simulink model "gm_uz_JL_invModel_PT1"  (R2025a)
settings: Solver=FixedStepDiscrete  StartTime=0.0  StopTime=10.0  RelTol=1e-3
settings Model: Creator=jonat  LastModifiedBy=jonat
settings SolverCC: AlgebraicLoopSolver=TrustRegion
settings DataIOCC: LimitDataPoints=on  SaveOutput=off  SaveTime=off
settings OptimizationCC: BlockReduction=off  ConditionallyExecuteInputs=off  DefaultParameterBehavior=Inlined  InheritOutputTypeSmallerThanSingle=on  LifeSpan=inf
settings DebuggingCC: AlgebraicLoopMsg=error  InheritedTsInSrcMsg=none  SingleTaskRateTransMsg=error  UnconnectedInputMsg=warning  UnconnectedOutputMsg=warning  UnconnectedLineMsg=warning  AllowSymbolicDim=off  StrictBusMsg=ErrorOnBusTreatedAsVector  SFUnexpectedBacktrackingDiag=warning  SFNoUnconditionalDefaultTransitionDiag=warning  SFExecutionAtInitializationDiag=none  ArithmeticOperatorsInVariantConditions=warning
settings HardwareCC: ProdBitPerPointer=32.0  ProdBitPerSizeT=32.0  ProdBitPerPtrDiffT=32.0  ProdLargestAtomicFloat=None  ProdIntDivRoundTo=Undefined  ProdEndianess=Unspecified  ProdWordSize=32.0  ProdHWDeviceType=ASIC/FPGA->ASIC/FPGA  ProdEqTarget=off
settings ModelReferenceCC: EnableRefExpFcnMdlSchedulingChecks=on
settings SFSimCC: SimUseLocalCustomCode=off  CustomCodeUndefinedFunction=UseInterfaceOnly
settings RTWCC: RTWUseLocalCustomCode=off  GPUComputeCapability=3.5
settings CodeAppCC: StateflowObjectComments=on
settings GRTTargetCC: TargetLangStandard=C89/C90 (ANSI)
settings ConfigComp: CovScope=ReferencedModels  CovMetricSettings=dw  CovSaveCumulativeToWorkspaceVar=on  CovSaveSingleToWorkspaceVar=on  CovExternalEMLEnable=off  CovSFcnEnable=off

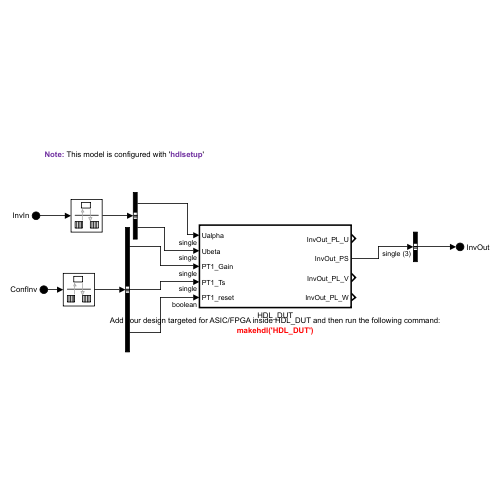
[thumbnail: Simulink's stored preview of the top-level diagram]
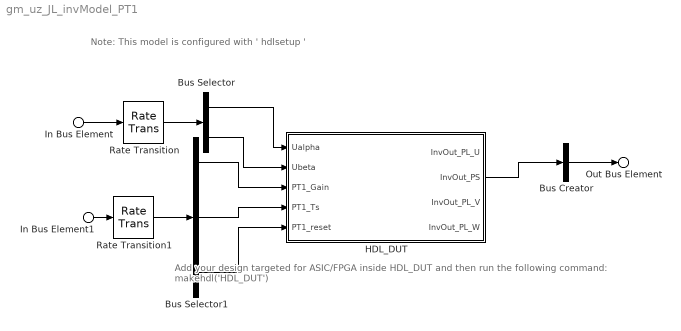
== system gm_uz_JL_invModel_PT1 ==
  note: Add your design targeted for ASIC/FPGA inside HDL_DUT and then run the following command:
      | makehdl('HDL_DUT')
  note: Note: This model is configured with ' hdlsetup '
  In Bus Element : Inport  PortName=InvIn
  In Bus Element1 : Inport  Port=2  PortName=ConfInv
  Bus Creator : BusCreator  Inputs=1  OutDataTypeStr=Bus: Bus_Inv_Out
      settings: InheritFromInputs=off
  Bus Selector : BusSelector  OutputSignals=Ualpha,Ubeta
  Bus Selector1 : BusSelector  OutputSignals=PT1_Gain,PT1_Ts,PT1_reset
  HDL_DUT : Subsystem  TreatAsAtomicUnit=on
  Rate Transition : RateTransition  OutPortSampleTime=1/1e6
  Rate Transition1 : RateTransition  OutPortSampleTime=1/1e6
  Out Bus Element : Outport  PortName=InvOut
  wires:
  Bus Selector1/3 -> HDL_DUT/5(PT1_reset)
  Bus Selector1/2 -> HDL_DUT/4(PT1_Ts)
  Bus Selector1/1 -> HDL_DUT/3(PT1_Gain)
  Bus Selector/2 -> HDL_DUT/2(Ubeta)
  Bus Selector/1 -> HDL_DUT/1(Ualpha)
  Bus Creator/1 -> Out Bus Element/1
  HDL_DUT/2(InvOut_PS) -> Bus Creator/1
  Rate Transition1/1 -> Bus Selector1/1
  Rate Transition/1 -> Bus Selector/1
  In Bus Element1/1 -> Rate Transition1/1
  In Bus Element/1 -> Rate Transition/1

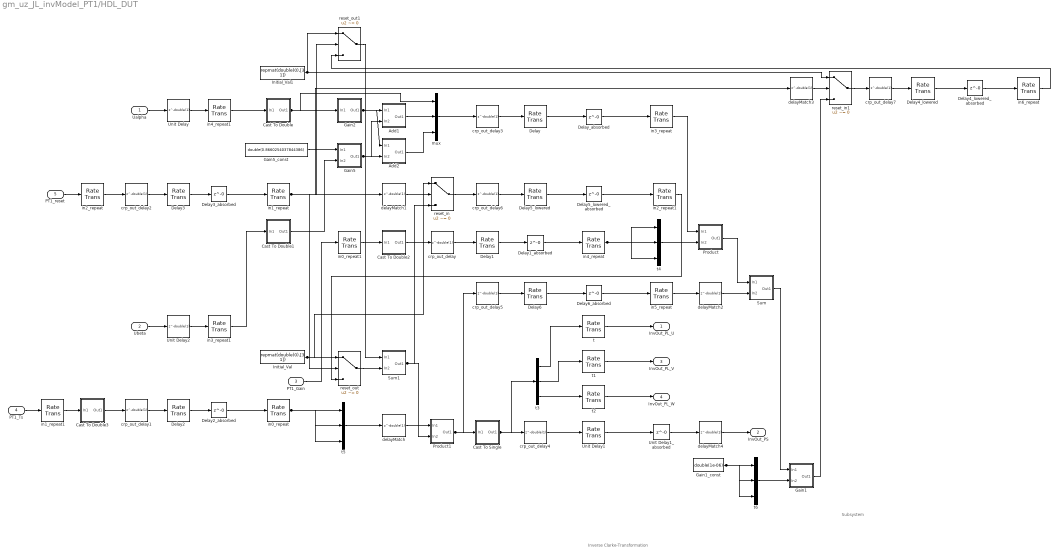
== system gm_uz_JL_invModel_PT1/HDL_DUT ==
  note: Subsystem
  note: Inverse Clarke-Transformation
  Ualpha : Inport  OutDataTypeStr=single  PortDimensions=1  SampleTime=1e-06
  Ubeta : Inport  Port=2  OutDataTypeStr=single  PortDimensions=1  SampleTime=1e-06
  PT1_Gain : Inport  Port=3  OutDataTypeStr=single  PortDimensions=1  SampleTime=1e-06
  PT1_Ts : Inport  Port=4  OutDataTypeStr=single  PortDimensions=1  SampleTime=1e-06
  PT1_reset : Inport  Port=5  OutDataTypeStr=boolean  PortDimensions=1  SampleTime=1e-06
  Add1 : Subsystem
      mask Display: disp('NFP\nadd');
  Add2 : Subsystem
      mask Display: disp('NFP\nadd');
  Cast To Double : Subsystem
      mask Display: disp('NFP\nconv');
  Cast To Double1 : Subsystem
      mask Display: disp('NFP\nconv');
  Cast To Double2 : Subsystem
      mask Display: disp('NFP\nconv');
  Cast To Double3 : Subsystem
      mask Display: disp('NFP\nconv');
  Cast To Single : Subsystem
      mask Display: disp('NFP\nconv');
  Delay{,1..3,6} (5 alike) : RateTransition  InitialCondition=double(0)  OutPortSampleTimeOpt=Multiple of input port sample time  OutPortSampleTimeMultiple=30
  Delay1_absorbed : Delay  DelayLength=0
  Delay2_absorbed : Delay  DelayLength=0
  Delay3_absorbed : Delay  DelayLength=0
  Delay4_lowered : RateTransition  InitialCondition=double(0)  OutPortSampleTimeOpt=Multiple of input port sample time  OutPortSampleTimeMultiple=30
  Delay4_lowered_absorbed : Delay  DelayLength=0
  Delay5_lowered : RateTransition  InitialCondition=double(0)  OutPortSampleTimeOpt=Multiple of input port sample time  OutPortSampleTimeMultiple=30
  Delay5_lowered_absorbed : Delay  DelayLength=0
  Delay6_absorbed : Delay  DelayLength=0
  Delay_absorbed : Delay  DelayLength=0
  Gain1 : Subsystem
      mask Display: disp('NFP\nmul');
  Gain1_const : Constant  Value=double(1e-06)  OutDataTypeStr=double  SampleTime=3.33333333333333e-08
  Gain2 : Subsystem
      mask Display: disp('NFP\ngain_pow2');
  Gain5 : Subsystem
      mask Display: disp('NFP\nmul');
  Gain5_const : Constant  Value=double(0.8660254037844386)  OutDataTypeStr=double  SampleTime=3.33333333333333e-08
  Initial_Val : Constant  Value="repmat(double(0),[3  1])"  OutDataTypeStr=double  SampleTime=3.33333333333333e-08
  Initial_Val1 : Constant  Value="repmat(double(0),[3  1])"  OutDataTypeStr=double  SampleTime=3.33333333333333e-08
  Product : Subsystem
      mask Display: disp('NFP\nmul');
  Product1 : Subsystem
      mask Display: disp('NFP\nmul');
  Sum : Subsystem
      mask Display: disp('NFP\nadd');
  Sum1 : Subsystem
      mask Display: disp('NFP\nadd');
  Unit Delay : Delay  DelayLength=double(1)  InitialCondition=0  SampleTime=1e-06
  Unit Delay1 : RateTransition  InitialCondition=double(0)  OutPortSampleTimeOpt=Multiple of input port sample time  OutPortSampleTimeMultiple=30
  Unit Delay1_absorbed : Delay  DelayLength=0
  Unit Delay2 : Delay  DelayLength=double(1)  InitialCondition=0  SampleTime=1e-06
  crp_out_delay{,1..7} (8 alike) : Delay  DelayLength=double(1)  InitialCondition=0  SampleTime=3.33333333333333e-08
  delayMatch{,1..3} (4 alike) : Delay  DelayLength=double(1)  InitialCondition=0  SampleTime=3.33333333333333e-08
  delayMatch4 : Delay  DelayLength=double(1)  InitialCondition=0  SampleTime=1e-06
  in0_repeat : RateTransition  Integrity=off  Deterministic=off  OutPortSampleTimeOpt=Multiple of input port sample time  OutPortSampleTimeMultiple=1/30
  in0_repeat1 : RateTransition  Integrity=off  Deterministic=off  OutPortSampleTimeOpt=Multiple of input port sample time  OutPortSampleTimeMultiple=1/30
  in1_repeat : RateTransition  Integrity=off  Deterministic=off  OutPortSampleTimeOpt=Multiple of input port sample time  OutPortSampleTimeMultiple=1/30
  in1_repeat1 : RateTransition  Integrity=off  Deterministic=off  OutPortSampleTimeOpt=Multiple of input port sample time  OutPortSampleTimeMultiple=1/30
  in2_repeat : RateTransition  Integrity=off  Deterministic=off  OutPortSampleTimeOpt=Multiple of input port sample time  OutPortSampleTimeMultiple=1/30
  in2_repeat1 : RateTransition  Integrity=off  Deterministic=off  OutPortSampleTimeOpt=Multiple of input port sample time  OutPortSampleTimeMultiple=1/30
  in3_repeat : RateTransition  Integrity=off  Deterministic=off  OutPortSampleTimeOpt=Multiple of input port sample time  OutPortSampleTimeMultiple=1/30
  in3_repeat1 : RateTransition  Integrity=off  Deterministic=off  OutPortSampleTimeOpt=Multiple of input port sample time  OutPortSampleTimeMultiple=1/30
  in4_repeat : RateTransition  Integrity=off  Deterministic=off  OutPortSampleTimeOpt=Multiple of input port sample time  OutPortSampleTimeMultiple=1/30
  in4_repeat1 : RateTransition  Integrity=off  Deterministic=off  OutPortSampleTimeOpt=Multiple of input port sample time  OutPortSampleTimeMultiple=1/30
  in5_repeat : RateTransition  Integrity=off  Deterministic=off  OutPortSampleTimeOpt=Multiple of input port sample time  OutPortSampleTimeMultiple=1/30
  in6_repeat : RateTransition  Integrity=off  Deterministic=off  OutPortSampleTimeOpt=Multiple of input port sample time  OutPortSampleTimeMultiple=1/30
  mux : Mux  Inputs=3
  reset_in : Switch  Criteria=u2 ~= 0  Threshold=double(0)  OutDataTypeStr=double  SampleTime=3.33333333333333e-08  SaturateOnIntegerOverflow=off  InputSameDT=off
  reset_in1 : Switch  Criteria=u2 ~= 0  Threshold=double(0)  OutDataTypeStr=double  SampleTime=3.33333333333333e-08  SaturateOnIntegerOverflow=off  InputSameDT=off
  reset_out : Switch  Criteria=u2 ~= 0  Threshold=double(0)  OutDataTypeStr=double  SampleTime=3.33333333333333e-08  SaturateOnIntegerOverflow=off  InputSameDT=off
  reset_out1 : Switch  Criteria=u2 ~= 0  Threshold=double(0)  OutDataTypeStr=double  SampleTime=3.33333333333333e-08  SaturateOnIntegerOverflow=off  InputSameDT=off
  t : RateTransition  InitialCondition=double(0)  OutPortSampleTimeOpt=Multiple of input port sample time  OutPortSampleTimeMultiple=30
  t1 : RateTransition  InitialCondition=double(0)  OutPortSampleTimeOpt=Multiple of input port sample time  OutPortSampleTimeMultiple=30
  t2 : RateTransition  InitialCondition=double(0)  OutPortSampleTimeOpt=Multiple of input port sample time  OutPortSampleTimeMultiple=30
  t3 : Demux  Outputs=3
  t4 : Mux  Inputs=3
  t5 : Mux  Inputs=3
  t6 : Mux  Inputs=3
  InvOut_PL_U : Outport  SampleTime=1e-06
  InvOut_PS : Outport  Port=2  SampleTime=1e-06
  InvOut_PL_V : Outport  Port=3  SampleTime=1e-06
  InvOut_PL_W : Outport  Port=4  SampleTime=1e-06
  wires:
  Delay/1 -> Delay_absorbed/1
  delayMatch/1 -> Product1/1(In1)
  reset_out/1 -> Sum1/2(In2)
  in1_repeat/1 -> delayMatch3/1, delayMatch1/1, reset_out1/2, reset_out/2
  PT1_Ts/1 -> in1_repeat1/1
  PT1_reset/1 -> in2_repeat/1
  crp_out_delay5/1 -> Delay6/1
  Delay5_lowered_absorbed/1 -> in2_repeat1/1
  in1_repeat1/1 -> Cast To Double3/1(In1)
  crp_out_delay6/1 -> Delay5_lowered/1
  crp_out_delay2/1 -> Delay3/1
  Delay6_absorbed/1 -> in5_repeat/1
  Gain5/1(Out1) -> Add1/2(In2), Add2/2(In2)
  Initial_Val1/1 -> reset_in1/1, reset_out1/1
  in2_repeat/1 -> crp_out_delay2/1
  Cast To Double3/1(Out1) -> crp_out_delay1/1
  Gain5_const/1 -> Gain5/1(In1)
  Ubeta/1 -> Unit Delay2/1
  reset_out1/1 -> Sum1/1(In1)
  Ualpha/1 -> Unit Delay/1
  crp_out_delay1/1 -> Delay2/1
  Delay2/1 -> Delay2_absorbed/1
  Unit Delay/1 -> in4_repeat1/1
  crp_out_delay3/1 -> Delay/1
  delayMatch1/1 -> reset_in/2
  Delay3/1 -> Delay3_absorbed/1
  crp_out_delay7/1 -> Delay4_lowered/1
  in0_repeat/1 -> t5/3, t5/2, t5/1
  Unit Delay2/1 -> in3_repeat1/1
  Delay_absorbed/1 -> in3_repeat/1
  in4_repeat1/1 -> Cast To Double/1(In1)
  Delay3_absorbed/1 -> in1_repeat/1
  in3_repeat1/1 -> Cast To Double1/1(In1)
  Delay2_absorbed/1 -> in0_repeat/1
  Cast To Double/1(Out1) -> Gain2/1(In1), mux/1
  mux/1 -> crp_out_delay3/1
  Cast To Double1/1(Out1) -> Gain5/2(In2)
  Cast To Double2/1(Out1) -> crp_out_delay/1
  t5/1 -> delayMatch/1
  Initial_Val/1 -> reset_in/1, reset_out/1
  Delay1/1 -> Delay1_absorbed/1
  reset_in/1 -> crp_out_delay6/1
  PT1_Gain/1 -> in0_repeat1/1
  Gain2/1(Out1) -> Add1/1(In1), Add2/1(In1)
  in0_repeat1/1 -> Cast To Double2/1(In1)
  Add1/1(Out1) -> mux/2
  in2_repeat1/1 -> reset_out/3
  Add2/1(Out1) -> mux/3
  Sum1/1(Out1) -> reset_in/3, Product1/2(In2)
  crp_out_delay4/1 -> Unit Delay1/1
  reset_in1/1 -> crp_out_delay7/1
  crp_out_delay/1 -> Delay1/1
  Product1/1(Out1) -> Cast To Single/1(In1), crp_out_delay5/1
  t/1 -> InvOut_PL_U/1
  Cast To Single/1(Out1) -> t3/1, crp_out_delay4/1
  Delay5_lowered/1 -> Delay5_lowered_absorbed/1
  Delay1_absorbed/1 -> in4_repeat/1
  Delay6/1 -> Delay6_absorbed/1
  t3/1 -> t/1
  t3/2 -> t1/1
  t1/1 -> InvOut_PL_V/1
  t3/3 -> t2/1
  in4_repeat/1 -> t4/3, t4/2, t4/1
  t2/1 -> InvOut_PL_W/1
  Unit Delay1/1 -> Unit Delay1_absorbed/1
  in3_repeat/1 -> Product/1(In1)
  t4/1 -> Product/2(In2)
  in5_repeat/1 -> delayMatch2/1
  Unit Delay1_absorbed/1 -> delayMatch4/1
  Product/1(Out1) -> Sum/1(In1)
  delayMatch2/1 -> Sum/2(In2)
  delayMatch4/1 -> InvOut_PS/1
  Gain1_const/1 -> t6/3, t6/2, t6/1
  Sum/1(Out1) -> Gain1/1(In1)
  t6/1 -> Gain1/2(In2)
  delayMatch3/1 -> reset_in1/2
  Gain1/1(Out1) -> reset_in1/3
  Delay4_lowered/1 -> Delay4_lowered_absorbed/1
  Delay4_lowered_absorbed/1 -> in6_repeat/1
  in6_repeat/1 -> reset_out1/3

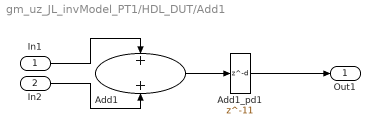
== system gm_uz_JL_invModel_PT1/HDL_DUT/Add1 ==
  In1 : Inport
  In2 : Inport  Port=2
  Add1 : Sum  OutDataTypeStr=double  SampleTime=3.33333333333333e-08
  Add1_pd1 : Delay  DelayLength=11
  Out1 : Outport
  wires:
  In1/1 -> Add1/1
  In2/1 -> Add1/2
  Add1/1 -> Add1_pd1/1
  Add1_pd1/1 -> Out1/1

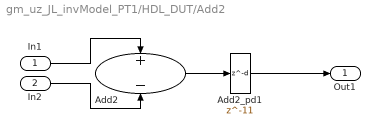
== system gm_uz_JL_invModel_PT1/HDL_DUT/Add2 ==
  In1 : Inport
  In2 : Inport  Port=2
  Add2 : Sum  Inputs=+-  OutDataTypeStr=double  SampleTime=3.33333333333333e-08
  Add2_pd1 : Delay  DelayLength=11
  Out1 : Outport
  wires:
  In1/1 -> Add2/1
  In2/1 -> Add2/2
  Add2/1 -> Add2_pd1/1
  Add2_pd1/1 -> Out1/1

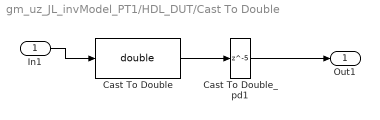
== system gm_uz_JL_invModel_PT1/HDL_DUT/Cast To Double ==
  In1 : Inport
  Cast To Double : DataTypeConversion  OutDataTypeStr=double  SampleTime=3.33333333333333e-08  SaturateOnIntegerOverflow=off  RndMeth=Floor
  Cast To Double_pd1 : Delay  DelayLength=5
  Out1 : Outport
  wires:
  In1/1 -> Cast To Double/1
  Cast To Double/1 -> Cast To Double_pd1/1
  Cast To Double_pd1/1 -> Out1/1

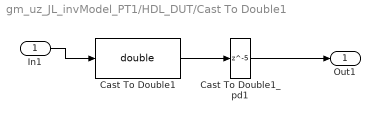
== system gm_uz_JL_invModel_PT1/HDL_DUT/Cast To Double1 ==
  In1 : Inport
  Cast To Double1 : DataTypeConversion  OutDataTypeStr=double  SampleTime=3.33333333333333e-08  SaturateOnIntegerOverflow=off  RndMeth=Floor
  Cast To Double1_pd1 : Delay  DelayLength=5
  Out1 : Outport
  wires:
  In1/1 -> Cast To Double1/1
  Cast To Double1/1 -> Cast To Double1_pd1/1
  Cast To Double1_pd1/1 -> Out1/1

== system gm_uz_JL_invModel_PT1/HDL_DUT/Cast To Double2 ==
  In1 : Inport
  Cast To Double2 : DataTypeConversion  OutDataTypeStr=double  SampleTime=3.33333333333333e-08  SaturateOnIntegerOverflow=off  RndMeth=Floor
  Cast To Double2_pd1 : Delay  DelayLength=5
  Out1 : Outport
  wires:
  In1/1 -> Cast To Double2/1
  Cast To Double2/1 -> Cast To Double2_pd1/1
  Cast To Double2_pd1/1 -> Out1/1

== system gm_uz_JL_invModel_PT1/HDL_DUT/Cast To Double3 ==
  In1 : Inport
  Cast To Double3 : DataTypeConversion  OutDataTypeStr=double  SampleTime=3.33333333333333e-08  SaturateOnIntegerOverflow=off  RndMeth=Floor
  Cast To Double3_pd1 : Delay  DelayLength=5
  Out1 : Outport
  wires:
  In1/1 -> Cast To Double3/1
  Cast To Double3/1 -> Cast To Double3_pd1/1
  Cast To Double3_pd1/1 -> Out1/1

== system gm_uz_JL_invModel_PT1/HDL_DUT/Cast To Single ==
  In1 : Inport
  Cast To Single : DataTypeConversion  OutDataTypeStr=single  SampleTime=3.33333333333333e-08  SaturateOnIntegerOverflow=off  RndMeth=Floor
  Cast To Single_pd1 : Delay  DelayLength=6
  Out1 : Outport
  wires:
  In1/1 -> Cast To Single/1
  Cast To Single/1 -> Cast To Single_pd1/1
  Cast To Single_pd1/1 -> Out1/1

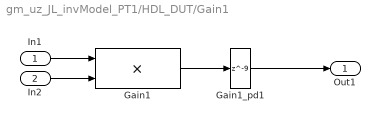
== system gm_uz_JL_invModel_PT1/HDL_DUT/Gain1 ==
  In1 : Inport
  In2 : Inport  Port=2
  Gain1 : Product  Inputs=**  OutDataTypeStr=double  SampleTime=3.33333333333333e-08
  Gain1_pd1 : Delay  DelayLength=9
  Out1 : Outport
  wires:
  In1/1 -> Gain1/1
  In2/1 -> Gain1/2
  Gain1/1 -> Gain1_pd1/1
  Gain1_pd1/1 -> Out1/1

== system gm_uz_JL_invModel_PT1/HDL_DUT/Gain2 ==
  In1 : Inport
  Gain2 : Gain  Gain=double(-0.5)
  Gain2_pd1 : Delay
  Out1 : Outport
  wires:
  In1/1 -> Gain2/1
  Gain2/1 -> Gain2_pd1/1
  Gain2_pd1/1 -> Out1/1

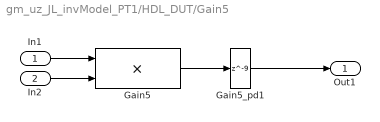
== system gm_uz_JL_invModel_PT1/HDL_DUT/Gain5 ==
  In1 : Inport
  In2 : Inport  Port=2
  Gain5 : Product  Inputs=**  OutDataTypeStr=double  SampleTime=3.33333333333333e-08
  Gain5_pd1 : Delay  DelayLength=9
  Out1 : Outport
  wires:
  In1/1 -> Gain5/1
  In2/1 -> Gain5/2
  Gain5/1 -> Gain5_pd1/1
  Gain5_pd1/1 -> Out1/1

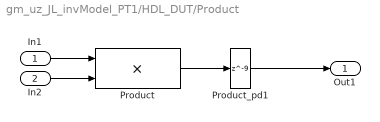
== system gm_uz_JL_invModel_PT1/HDL_DUT/Product ==
  In1 : Inport
  In2 : Inport  Port=2
  Product : Product  Inputs=**  OutDataTypeStr=double  SampleTime=3.33333333333333e-08
  Product_pd1 : Delay  DelayLength=9
  Out1 : Outport
  wires:
  In1/1 -> Product/1
  In2/1 -> Product/2
  Product/1 -> Product_pd1/1
  Product_pd1/1 -> Out1/1

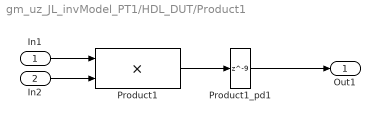
== system gm_uz_JL_invModel_PT1/HDL_DUT/Product1 ==
  In1 : Inport
  In2 : Inport  Port=2
  Product1 : Product  Inputs=**  OutDataTypeStr=double  SampleTime=3.33333333333333e-08
  Product1_pd1 : Delay  DelayLength=9
  Out1 : Outport
  wires:
  In1/1 -> Product1/1
  In2/1 -> Product1/2
  Product1/1 -> Product1_pd1/1
  Product1_pd1/1 -> Out1/1

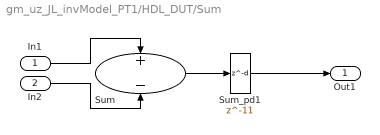
== system gm_uz_JL_invModel_PT1/HDL_DUT/Sum ==
  In1 : Inport
  In2 : Inport  Port=2
  Sum : Sum  Inputs=+-  OutDataTypeStr=double  SampleTime=3.33333333333333e-08
  Sum_pd1 : Delay  DelayLength=11
  Out1 : Outport
  wires:
  In1/1 -> Sum/1
  In2/1 -> Sum/2
  Sum/1 -> Sum_pd1/1
  Sum_pd1/1 -> Out1/1

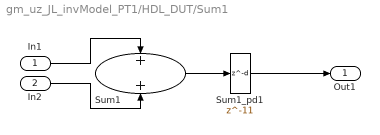
== system gm_uz_JL_invModel_PT1/HDL_DUT/Sum1 ==
  In1 : Inport
  In2 : Inport  Port=2
  Sum1 : Sum  OutDataTypeStr=double  SampleTime=3.33333333333333e-08
  Sum1_pd1 : Delay  DelayLength=11
  Out1 : Outport
  wires:
  In1/1 -> Sum1/1
  In2/1 -> Sum1/2
  Sum1/1 -> Sum1_pd1/1
  Sum1_pd1/1 -> Out1/1
